simulink model "test_s_func"  (R2018a)
settings: Solver=VariableStepAuto  StartTime=0.0  StopTime=20/10000  RelTol=1e-3
settings Model: Creator=facu  LastModifiedBy=facu

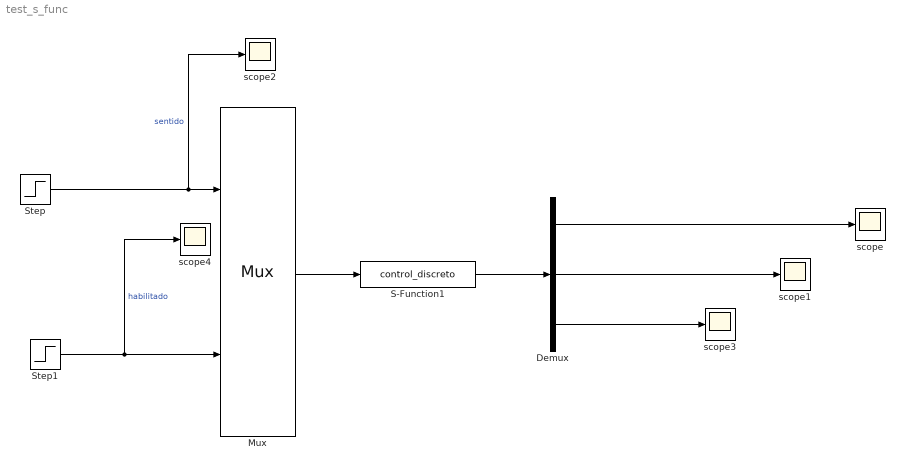
== system test_s_func ==
  Demux : Demux  Outputs=3
  Mux : Mux  Inputs=2
      settings: DisplayOption=signals
  S-Function1 : S-Function  FunctionName=control_discreto  SFunctionDeploymentMode=off  EnableBusSupport=off
  Step : Step  Time=10/10000  SampleTime=1/10000
  Step1 : Step  Time=3/10000  SampleTime=1/10000
  scope{,1..4} (5 alike) : Scope
  wires:
  S-Function1/1 -> Demux/1
  Step/1 -> scope2/1, Mux/1  "sentido"
  Mux/1 -> S-Function1/1
  Demux/1 -> scope/1
  Demux/2 -> scope1/1
  Demux/3 -> scope3/1
  Step1/1 -> scope4/1, Mux/2  "habilitado"
